simulink subsystem "INDI_Controller_PQR"  (R2023b)
settings: Solver=VariableStepAuto  StartTime=0.0  StopTime=10.0  RelTol=1e-3
undefined symbols (not defined in the file): controlDeflections, dataBase, deltaLEF
libraries: aerolibutil x1, simulink_extras x1
settings Model: Creator=cyber  LastModifiedBy=cyber

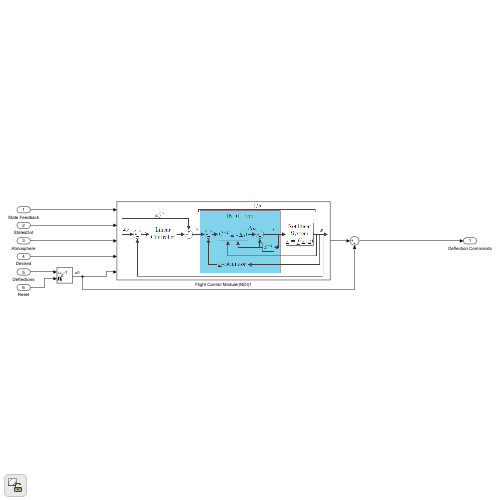
[thumbnail: Simulink's stored preview of the top-level diagram]
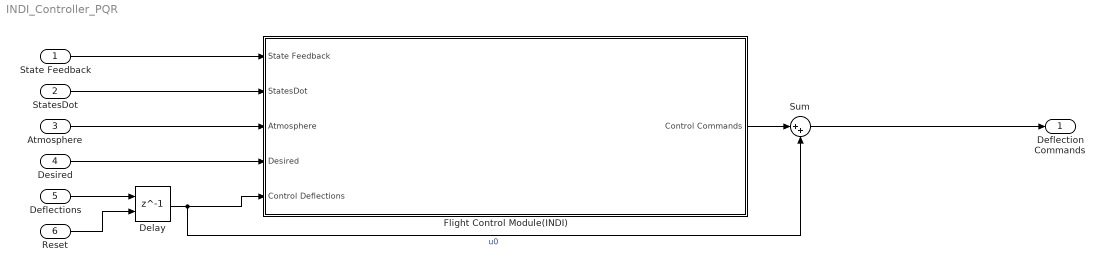
== system INDI_Controller_PQR ==
  State Feedback : Inport
  StatesDot : Inport  Port=2
  Atmosphere : Inport  Port=3
  Desired : Inport  Port=4
  Deflections : Inport  Port=5
  Reset : Inport  Port=6
  Delay : Delay  DelayLength=1  InitialCondition=[controlDeflections(1); controlDeflections(2); controlDeflections(3); controlDeflections(4); deltaLEF; 0]  ExternalReset=Either
      settings: InputPortMap=u0,r5
  Flight Control Module(INDI) : Subsystem
      mask Display: image('INDI.png'); % Use "Edit Image" on toolstrip to change.
  Sum : Sum  Inputs=|++
  Deflection Commands : Outport
  wires:
  Sum/1 -> Deflection Commands/1
  Flight Control Module(INDI)/1(Control Commands) -> Sum/1
  Reset/1 -> Delay/2
  Delay/1 -> Flight Control Module(INDI)/5(Control Deflections), Sum/2  "u0"
  Atmosphere/1 -> Flight Control Module(INDI)/3(Atmosphere)
  StatesDot/1 -> Flight Control Module(INDI)/2(StatesDot)
  State Feedback/1 -> Flight Control Module(INDI)/1(State Feedback)
  Deflections/1 -> Delay/1
  Desired/1 -> Flight Control Module(INDI)/4(Desired)

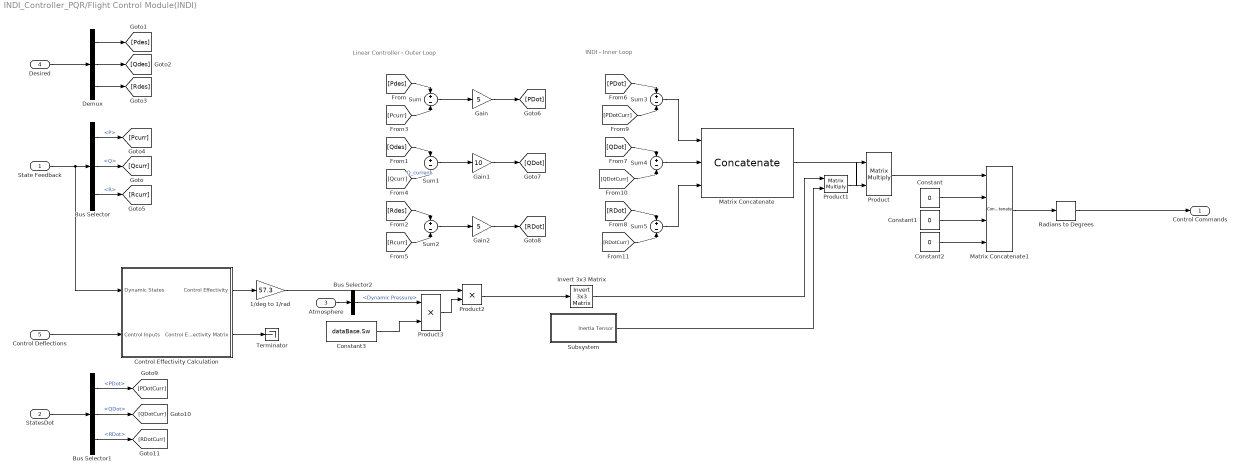
== system INDI_Controller_PQR/Flight Control Module(INDI) ==
  note: INDI - Inner Loop
  note: Linear Controller - Outer Loop
  State Feedback : Inport
  StatesDot : Inport  Port=2
  Atmosphere : Inport  Port=3
  Desired : Inport  Port=4
  Control Deflections : Inport  Port=5
  1/deg to 1/rad : Gain  Gain=57.3
  Bus Selector : BusSelector  OutputSignals=P,Q,R
  Bus Selector1 : BusSelector  OutputSignals=PDot,QDot,RDot
  Bus Selector2 : BusSelector  OutputSignals=Dynamic Pressure
  Constant : Constant  Value=0
  Constant1 : Constant  Value=0
  Constant2 : Constant  Value=0
  Constant3 : Constant  Value=dataBase.Sw
  Control Effectivity Calculation : Subsystem
      mask Display: image('F16.PNG'); % Use "Edit Image" on toolstrip to change.
  Demux : Demux  Outputs=3
  Gain : Gain  Gain=5
  Gain1 : Gain  Gain=10
  Gain2 : Gain  Gain=5
  Invert 3x3 Matrix : aerolibutil/Invert  3x3 Matrix
  Matrix Concatenate : Concatenate  NumInputs=3  Mode=Multidimensional array
  Matrix Concatenate1 : Concatenate  NumInputs=4  Mode=Multidimensional array
  Product : Product  Multiplication=Matrix(*)
  Product1 : Product  Multiplication=Matrix(*)
  Product2 : Product
  Product3 : Product
  Radians to Degrees : simulink_extras/Transformations/Radians to Degrees
  Subsystem : Subsystem
  Sum{,1..5} (6 alike) : Sum  Inputs=+|-
  Terminator : Terminator
  Control Commands : Outport
  wires:
  State Feedback/1 -> Control Effectivity Calculation/1(Dynamic States), Bus Selector/1
  Bus Selector/2 -> [Qcurr]  "<Q>"
  Desired/1 -> Demux/1
  Demux/1 -> [Pdes]
  Demux/2 -> [Qdes]
  Demux/3 -> [Rdes]
  Control Deflections/1 -> Control Effectivity Calculation/2(Control Inputs)
  Bus Selector/1 -> [Pcurr]  "<P>"
  Bus Selector/3 -> [Rcurr]  "<R>"
  [Pdes] -> Sum/1
  [Pcurr] -> Sum/2
  Sum/1 -> Gain/1
  [Qdes] -> Sum1/1
  [Qcurr] -> Sum1/2  "Q_current"
  Sum1/1 -> Gain1/1
  [Rdes] -> Sum2/1
  [Rcurr] -> Sum2/2
  Sum2/1 -> Gain2/1
  Gain/1 -> [PDot]
  Gain1/1 -> [QDot]
  Gain2/1 -> [RDot]
  StatesDot/1 -> Bus Selector1/1
  [PDot] -> Sum3/1
  [PDotCurr] -> Sum3/2
  [QDot] -> Sum4/1
  [QDotCurr] -> Sum4/2
  [RDot] -> Sum5/1
  [RDotCurr] -> Sum5/2
  Sum3/1 -> Matrix Concatenate/1
  Sum4/1 -> Matrix Concatenate/2
  Sum5/1 -> Matrix Concatenate/3
  Matrix Concatenate/1 -> Product/2
  Control Effectivity Calculation/1(Control Effectivity) -> 1/deg to 1/rad/1
  Product1/1 -> Product/1
  Constant/1 -> Matrix Concatenate1/2
  Constant1/1 -> Matrix Concatenate1/3
  Constant2/1 -> Matrix Concatenate1/4
  Matrix Concatenate1/1 -> Radians to Degrees/1
  Product/1 -> Matrix Concatenate1/1
  Radians to Degrees/1 -> Control Commands/1
  Bus Selector1/3 -> [RDotCurr]  "<RDot>"
  Bus Selector1/2 -> [QDotCurr]  "<QDot>"
  Bus Selector1/1 -> [PDotCurr]  "<PDot>"
  1/deg to 1/rad/1 -> Product2/1
  Product2/1 -> Invert 3x3 Matrix/1
  Atmosphere/1 -> Bus Selector2/1
  Product3/1 -> Product2/2
  Constant3/1 -> Product3/2
  Invert 3x3 Matrix/1 -> Product1/1
  Subsystem/1(Inertia Tensor) -> Product1/2
  Bus Selector2/1 -> Product3/1  "<Dynamic Pressure>"
  Control Effectivity Calculation/2(Control Effectivity Matrix) -> Terminator/1

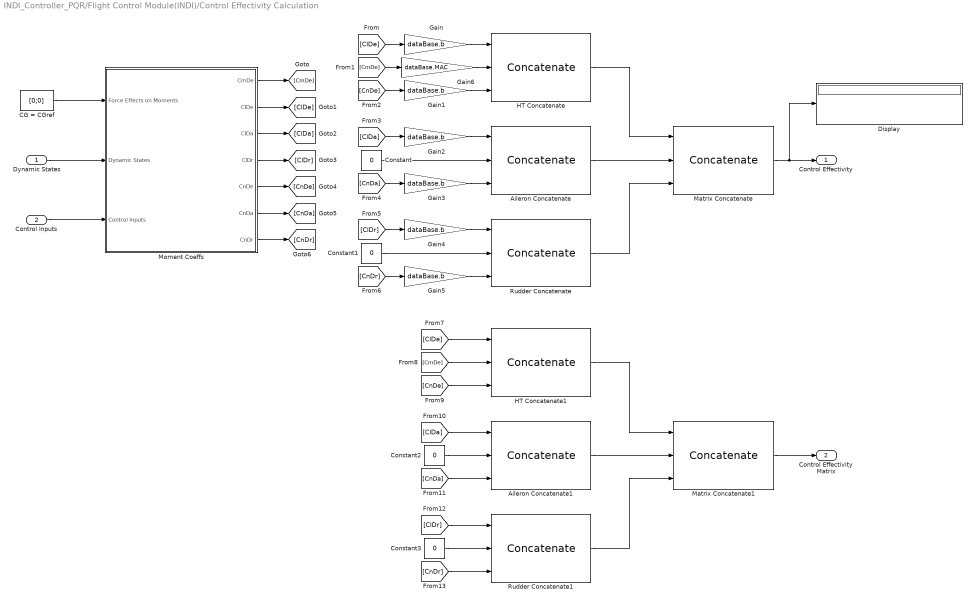
== system INDI_Controller_PQR/Flight Control Module(INDI)/Control Effectivity Calculation ==
  Dynamic States : Inport
  Control Inputs : Inport  Port=2
  Aileron Concatenate : Concatenate  NumInputs=3  Mode=Multidimensional array
  Aileron Concatenate1 : Concatenate  NumInputs=3  Mode=Multidimensional array
  CG = CGref : Constant  Value=[0;0]
  Constant{,1..3} (4 alike) : Constant  Value=0
  Display : Display
  Gain{,1..5} (6 alike) : Gain  Gain=dataBase.b
  Gain6 : Gain  Gain=dataBase.MAC
  HT Concatenate : Concatenate  NumInputs=3  Mode=Multidimensional array
  HT Concatenate1 : Concatenate  NumInputs=3  Mode=Multidimensional array
  Matrix Concatenate : Concatenate  NumInputs=3  Mode=Multidimensional array  ConcatenateDimension=2
  Matrix Concatenate1 : Concatenate  NumInputs=3  Mode=Multidimensional array  ConcatenateDimension=2
  Moment Coeffs : Subsystem
  Rudder Concatenate : Concatenate  NumInputs=3  Mode=Multidimensional array
  Rudder Concatenate1 : Concatenate  NumInputs=3  Mode=Multidimensional array
  Control Effectivity : Outport
  Control Effectivity Matrix : Outport  Port=2
  wires:
  Dynamic States/1 -> Moment Coeffs/2(Dynamic States)
  Control Inputs/1 -> Moment Coeffs/3(Control Inputs)
  CG = CGref/1 -> Moment Coeffs/1(Force Effects on Moments)
  Moment Coeffs/1(" CmDe") -> [CmDe]
  Moment Coeffs/2(" ClDe") -> [ClDe]
  Moment Coeffs/3(" ClDa") -> [ClDa]
  Moment Coeffs/4(" ClDr") -> [ClDr]
  Moment Coeffs/5(CnDe) -> [CnDe]
  Moment Coeffs/6(CnDa) -> [CnDa]
  Moment Coeffs/7(CnDr) -> [CnDr]
  HT Concatenate/1 -> Matrix Concatenate/1
  Aileron Concatenate/1 -> Matrix Concatenate/2
  Rudder Concatenate/1 -> Matrix Concatenate/3
  [ClDe] -> Gain/1
  [CmDe] -> Gain6/1
  [CnDe] -> Gain1/1
  [ClDa] -> Gain2/1
  Constant/1 -> Aileron Concatenate/2
  [CnDa] -> Gain3/1
  [ClDr] -> Gain4/1
  [CnDr] -> Gain5/1
  Constant1/1 -> Rudder Concatenate/2
  Matrix Concatenate/1 -> Display/1, Control Effectivity/1
  Gain/1 -> HT Concatenate/1
  Gain1/1 -> HT Concatenate/3
  Gain2/1 -> Aileron Concatenate/1
  Gain3/1 -> Aileron Concatenate/3
  Gain4/1 -> Rudder Concatenate/1
  Gain5/1 -> Rudder Concatenate/3
  Gain6/1 -> HT Concatenate/2
  [CmDe] -> HT Concatenate1/2
  [ClDe] -> HT Concatenate1/1
  [CnDa] -> Aileron Concatenate1/3
  [CnDe] -> HT Concatenate1/3
  [ClDa] -> Aileron Concatenate1/1
  Rudder Concatenate1/1 -> Matrix Concatenate1/3
  Matrix Concatenate1/1 -> Control Effectivity Matrix/1
  [ClDr] -> Rudder Concatenate1/1
  HT Concatenate1/1 -> Matrix Concatenate1/1
  [CnDr] -> Rudder Concatenate1/3
  Aileron Concatenate1/1 -> Matrix Concatenate1/2
  Constant2/1 -> Aileron Concatenate1/2
  Constant3/1 -> Rudder Concatenate1/2

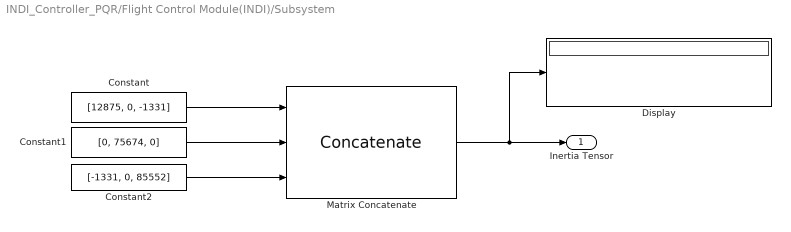
== system INDI_Controller_PQR/Flight Control Module(INDI)/Subsystem ==
  Constant : Constant  Value=[12875, 0, -1331]
  Constant1 : Constant  Value=[0, 75674, 0]
  Constant2 : Constant  Value=[-1331, 0, 85552]
  Display : Display
  Matrix Concatenate : Concatenate  NumInputs=3  Mode=Multidimensional array  ConcatenateDimension=2
  Inertia Tensor : Outport
  wires:
  Constant/1 -> Matrix Concatenate/1
  Constant2/1 -> Matrix Concatenate/3
  Constant1/1 -> Matrix Concatenate/2
  Matrix Concatenate/1 -> Display/1, Inertia Tensor/1

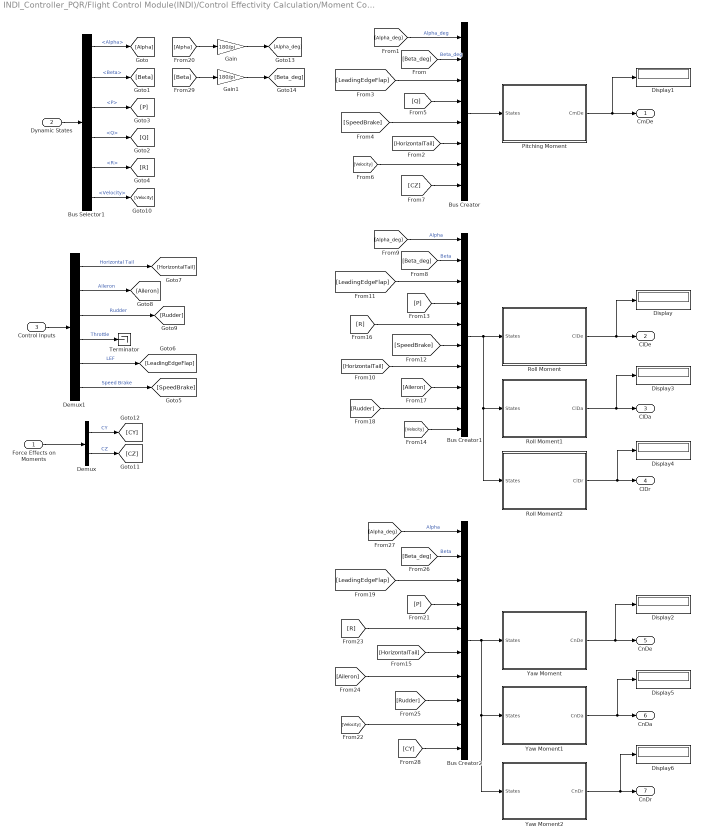
== system INDI_Controller_PQR/Flight Control Module(INDI)/Control Effectivity Calculation/Moment Coeffs ==
  Force Effects on Moments : Inport
  Dynamic States : Inport  Port=2
  Control Inputs : Inport  Port=3
  Bus Creator : BusCreator  Inputs=8
  Bus Creator1 : BusCreator  Inputs=10
  Bus Creator2 : BusCreator  Inputs=10
  Bus Selector1 : BusSelector  OutputSignals=Alpha,Beta,P,Q,R,Velocity
  Demux : Demux  Outputs=2
  Demux1 : Demux  Outputs=6
  Display{,1..6} (7 alike) : Display
  Gain : Gain  Gain=180/pi
  Gain1 : Gain  Gain=180/pi
  Pitching Moment : Subsystem
  Roll Moment : Subsystem
  Roll Moment1 : Subsystem
  Roll Moment2 : Subsystem
  Terminator : Terminator
  Yaw Moment : Subsystem
  Yaw Moment1 : Subsystem
  Yaw Moment2 : Subsystem
  " CmDe" : Outport
  " ClDe" : Outport  Port=2
  " ClDa" : Outport  Port=3
  " ClDr" : Outport  Port=4
  CnDe : Outport  Port=5
  CnDa : Outport  Port=6
  CnDr : Outport  Port=7
  wires:
  Pitching Moment/1(CmDe) -> Display1/1, " CmDe"/1
  Bus Creator/1 -> Pitching Moment/1(States)
  [SpeedBrake] -> Bus Creator/5
  [LeadingEdgeFlap] -> Bus Creator/3
  [Q] -> Bus Creator/4
  [HorizontalTail] -> Bus Creator/6
  [Velocity] -> Bus Creator/7
  [CZ] -> Bus Creator/8
  Force Effects on Moments/1 -> Demux/1
  Demux/1 -> [CY]  "CY"
  Demux/2 -> [CZ]  "CZ"
  [P] -> Bus Creator1/4
  [LeadingEdgeFlap] -> Bus Creator1/3
  Roll Moment/1(ClDe) -> Display/1, " ClDe"/1
  [Velocity] -> Bus Creator1/10
  [R] -> Bus Creator1/5
  [SpeedBrake] -> Bus Creator1/6
  [HorizontalTail] -> Bus Creator1/7
  [Aileron] -> Bus Creator1/8
  [Rudder] -> Bus Creator1/9
  [Rudder] -> Bus Creator2/8
  [Aileron] -> Bus Creator2/7
  [HorizontalTail] -> Bus Creator2/6
  [R] -> Bus Creator2/5
  [Velocity] -> Bus Creator2/9
  [LeadingEdgeFlap] -> Bus Creator2/3
  [P] -> Bus Creator2/4
  Bus Creator2/1 -> Yaw Moment2/1(States), Yaw Moment1/1(States), Yaw Moment/1(States)
  Bus Selector1/4 -> [Q]  "<Q>"
  Demux1/1 -> [HorizontalTail]  "Horizontal Tail"
  Control Inputs/1 -> Demux1/1
  Demux1/6 -> [SpeedBrake]  "Speed Brake"
  Demux1/2 -> [Aileron]  "Aileron"
  Bus Selector1/6 -> [Velocity]  "<Velocity>"
  Bus Selector1/3 -> [P]  "<P>"
  Bus Selector1/2 -> [Beta]  "<Beta>"
  Demux1/3 -> [Rudder]  "Rudder"
  Bus Selector1/5 -> [R]  "<R>"
  Demux1/5 -> [LeadingEdgeFlap]  "LEF"
  Dynamic States/1 -> Bus Selector1/1
  Bus Selector1/1 -> [Alpha]  "<Alpha>"
  Bus Creator1/1 -> Roll Moment2/1(States), Roll Moment1/1(States), Roll Moment/1(States)
  Gain1/1 -> [Beta_deg]
  [Beta] -> Gain1/1
  [Alpha] -> Gain/1
  Gain/1 -> [Alpha_deg]
  [Alpha_deg] -> Bus Creator/1  "Alpha_deg"
  [Beta_deg] -> Bus Creator/2  "Beta_deg"
  [Alpha_deg] -> Bus Creator1/1  "Alpha"
  [Beta_deg] -> Bus Creator1/2  "Beta"
  [Alpha_deg] -> Bus Creator2/1  "Alpha"
  [Beta_deg] -> Bus Creator2/2  "Beta"
  [CY] -> Bus Creator2/10
  Roll Moment1/1(ClDa) -> Display3/1, " ClDa"/1
  Roll Moment2/1(ClDr) -> Display4/1, " ClDr"/1
  Yaw Moment/1(CnDe) -> CnDe/1, Display2/1
  Yaw Moment1/1(CnDa) -> Display5/1, CnDa/1
  Yaw Moment2/1(CnDr) -> Display6/1, CnDr/1
  Demux1/4 -> Terminator/1  "Throttle"

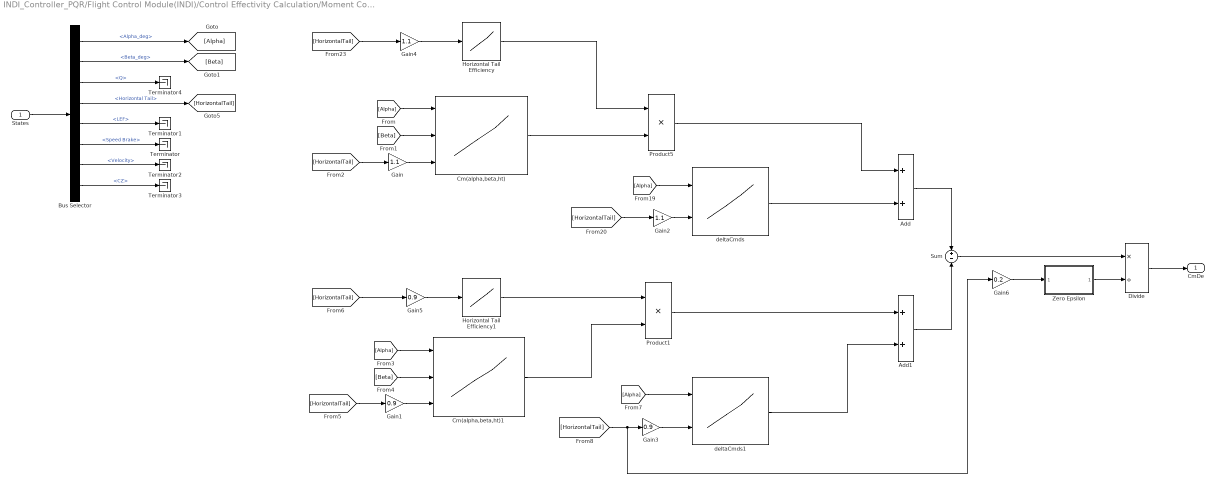
== system INDI_Controller_PQR/Flight Control Module(INDI)/Control Effectivity Calculation/Moment Coeffs/Pitching Moment ==
  States : Inport
  Add : Sum
  Add1 : Sum
  Bus Selector : BusSelector  OutputSignals=Alpha_deg,Beta_deg,Q,Horizontal Tail,LEF,Speed Brake,Velocity,CZ
  Cm(alpha,beta,ht) : Lookup_n-D  NumberOfTableDimensions=3  BreakpointsForDimension1=dataBase.f16_AerodynamicData.BP.Cm.Cm.alpha  BreakpointsForDimension2=dataBase.f16_AerodynamicData.BP.Cm.Cm.beta  BreakpointsForDimension3=dataBase.f16_AerodynamicData.BP.Cm.Cm.dHT  Table=dataBase.f16_AerodynamicData.data.Cm.Cm  ExtrapMethod=Clip  InternalRulePriority=Speed  RndMeth=Simplest
      settings: InputPortMap=u0,u1,u2
  Cm(alpha,beta,ht)1 : Lookup_n-D  NumberOfTableDimensions=3  BreakpointsForDimension1=dataBase.f16_AerodynamicData.BP.Cm.Cm.alpha  BreakpointsForDimension2=dataBase.f16_AerodynamicData.BP.Cm.Cm.beta  BreakpointsForDimension3=dataBase.f16_AerodynamicData.BP.Cm.Cm.dHT  Table=dataBase.f16_AerodynamicData.data.Cm.Cm  ExtrapMethod=Clip  InternalRulePriority=Speed  RndMeth=Simplest
      settings: InputPortMap=u0,u1,u2
  Divide : Product  Inputs=*/
  Gain : Gain  Gain=1.1
  Gain1 : Gain  Gain=0.9
  Gain2 : Gain  Gain=1.1
  Gain3 : Gain  Gain=0.9
  Gain4 : Gain  Gain=1.1
  Gain5 : Gain  Gain=0.9
  Gain6 : Gain  Gain=0.2
  Horizontal Tail Efficiency : Lookup_n-D  NumberOfTableDimensions=1  BreakpointsForDimension1=dataBase.f16_AerodynamicData.BP.Cm.n_dHT.dHT  Table=dataBase.f16_AerodynamicData.data.Cm.n_dHT  ExtrapMethod=Clip  InternalRulePriority=Speed  RndMeth=Simplest
  Horizontal Tail Efficiency1 : Lookup_n-D  NumberOfTableDimensions=1  BreakpointsForDimension1=dataBase.f16_AerodynamicData.BP.Cm.n_dHT.dHT  Table=dataBase.f16_AerodynamicData.data.Cm.n_dHT  ExtrapMethod=Clip  InternalRulePriority=Speed  RndMeth=Simplest
  Product1 : Product
  Product5 : Product
  Sum : Sum  Inputs=+|-
  Terminator{,1..4} (5 alike) : Terminator
  Zero Epsilon : Subsystem  ReferencedSubsystem=Zero_Epsilon
  deltaCmds : Lookup_n-D  BreakpointsForDimension1=dataBase.f16_AerodynamicData.BP.Cm.deltaCmds.alpha  BreakpointsForDimension2=dataBase.f16_AerodynamicData.BP.Cm.deltaCmds.dHT  Table=dataBase.f16_AerodynamicData.data.Cm.deltaCmds  ExtrapMethod=Clip  InternalRulePriority=Speed  RndMeth=Simplest
      settings: InputPortMap=u0,u1
  deltaCmds1 : Lookup_n-D  BreakpointsForDimension1=dataBase.f16_AerodynamicData.BP.Cm.deltaCmds.alpha  BreakpointsForDimension2=dataBase.f16_AerodynamicData.BP.Cm.deltaCmds.dHT  Table=dataBase.f16_AerodynamicData.data.Cm.deltaCmds  ExtrapMethod=Clip  InternalRulePriority=Speed  RndMeth=Simplest
      settings: InputPortMap=u0,u1
  CmDe : Outport
  wires:
  Zero Epsilon/1 -> Divide/2
  Gain6/1 -> Zero Epsilon/1
  [Alpha] -> Cm(alpha,beta,ht)/1
  States/1 -> Bus Selector/1
  [Beta] -> Cm(alpha,beta,ht)/2
  [Alpha] -> deltaCmds/1
  Product5/1 -> Add/1
  Cm(alpha,beta,ht)/1 -> Product5/2
  Horizontal Tail Efficiency/1 -> Product5/1
  Bus Selector/1 -> [Alpha]  "<Alpha_deg>"
  Bus Selector/2 -> [Beta]  "<Beta_deg>"
  Bus Selector/3 -> Terminator4/1  "<Q>"
  Bus Selector/4 -> [HorizontalTail]  "<Horizontal Tail>"
  Bus Selector/5 -> Terminator1/1  "<LEF>"
  Bus Selector/6 -> Terminator/1  "<Speed Brake>"
  Bus Selector/7 -> Terminator2/1  "<Velocity>"
  Bus Selector/8 -> Terminator3/1  "<CZ>"
  [HorizontalTail] -> Gain/1
  Gain/1 -> Cm(alpha,beta,ht)/3
  [HorizontalTail] -> Gain2/1
  Gain2/1 -> deltaCmds/2
  Add/1 -> Sum/1
  [HorizontalTail] -> Gain1/1
  Gain1/1 -> Cm(alpha,beta,ht)1/3
  [Beta] -> Cm(alpha,beta,ht)1/2
  Horizontal Tail Efficiency1/1 -> Product1/1
  [Alpha] -> Cm(alpha,beta,ht)1/1
  Cm(alpha,beta,ht)1/1 -> Product1/2
  [HorizontalTail] -> Gain3/1, Gain6/1
  Gain3/1 -> deltaCmds1/2
  [Alpha] -> deltaCmds1/1
  Product1/1 -> Add1/1
  deltaCmds1/1 -> Add1/2
  Add1/1 -> Sum/2
  deltaCmds/1 -> Add/2
  Sum/1 -> Divide/1
  Divide/1 -> CmDe/1
  [HorizontalTail] -> Gain4/1
  Gain4/1 -> Horizontal Tail Efficiency/1
  [HorizontalTail] -> Gain5/1
  Gain5/1 -> Horizontal Tail Efficiency1/1

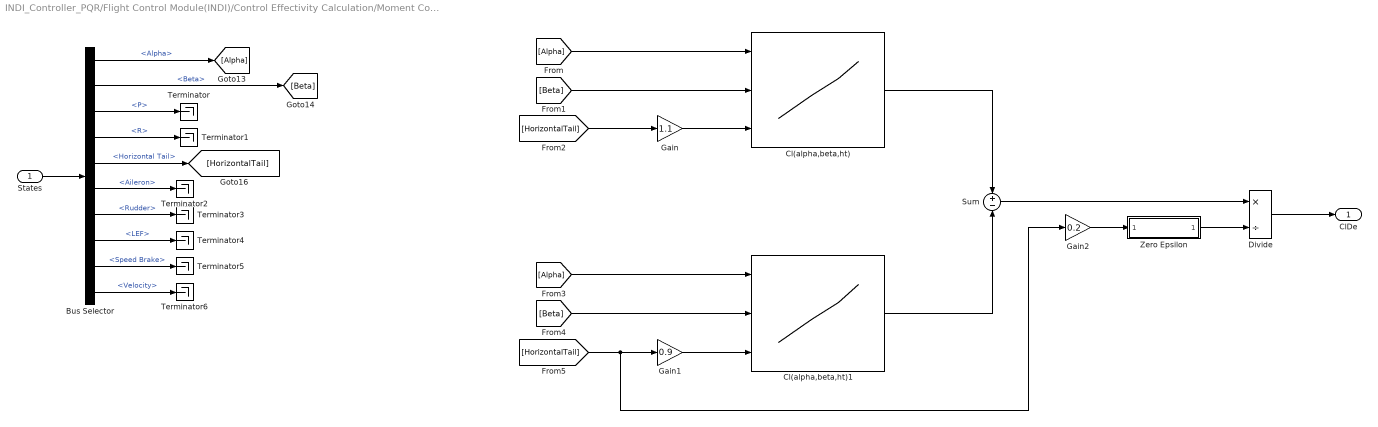
== system INDI_Controller_PQR/Flight Control Module(INDI)/Control Effectivity Calculation/Moment Coeffs/Roll Moment ==
  States : Inport
  Bus Selector : BusSelector  OutputSignals=Alpha,Beta,P,R,Horizontal Tail,Aileron,Rudder,LEF,Speed Brake,Velocity
  Cl(alpha,beta,ht) : Lookup_n-D  NumberOfTableDimensions=3  BreakpointsForDimension1=dataBase.f16_AerodynamicData.BP.Cl.Cl.alpha  BreakpointsForDimension2=dataBase.f16_AerodynamicData.BP.Cl.Cl.beta  BreakpointsForDimension3=dataBase.f16_AerodynamicData.BP.Cl.Cl.dHT  Table=dataBase.f16_AerodynamicData.data.Cl.Cl  ExtrapMethod=Clip  InternalRulePriority=Speed  RndMeth=Simplest
      settings: InputPortMap=u0,u1,u2
  Cl(alpha,beta,ht)1 : Lookup_n-D  NumberOfTableDimensions=3  BreakpointsForDimension1=dataBase.f16_AerodynamicData.BP.Cl.Cl.alpha  BreakpointsForDimension2=dataBase.f16_AerodynamicData.BP.Cl.Cl.beta  BreakpointsForDimension3=dataBase.f16_AerodynamicData.BP.Cl.Cl.dHT  Table=dataBase.f16_AerodynamicData.data.Cl.Cl  ExtrapMethod=Clip  InternalRulePriority=Speed  RndMeth=Simplest
      settings: InputPortMap=u0,u1,u2
  Divide : Product  Inputs=*/
  Gain : Gain  Gain=1.1
  Gain1 : Gain  Gain=0.9
  Gain2 : Gain  Gain=0.2
  Sum : Sum  Inputs=+|-
  Terminator{,1..6} (7 alike) : Terminator
  Zero Epsilon : Subsystem  ReferencedSubsystem=Zero_Epsilon
  ClDe : Outport
  wires:
  Zero Epsilon/1 -> Divide/2
  Gain2/1 -> Zero Epsilon/1
  Cl(alpha,beta,ht)/1 -> Sum/1
  [Alpha] -> Cl(alpha,beta,ht)/1
  [Beta] -> Cl(alpha,beta,ht)/2
  Bus Selector/5 -> [HorizontalTail]  "<Horizontal Tail>"
  States/1 -> Bus Selector/1
  Bus Selector/2 -> [Beta]  "<Beta>"
  Bus Selector/1 -> [Alpha]  "<Alpha>"
  [Alpha] -> Cl(alpha,beta,ht)1/1
  [Beta] -> Cl(alpha,beta,ht)1/2
  Cl(alpha,beta,ht)1/1 -> Sum/2
  [HorizontalTail] -> Gain/1
  Gain/1 -> Cl(alpha,beta,ht)/3
  [HorizontalTail] -> Gain2/1, Gain1/1
  Gain1/1 -> Cl(alpha,beta,ht)1/3
  Sum/1 -> Divide/1
  Divide/1 -> ClDe/1
  Bus Selector/3 -> Terminator/1  "<P>"
  Bus Selector/4 -> Terminator1/1  "<R>"
  Bus Selector/6 -> Terminator2/1  "<Aileron>"
  Bus Selector/7 -> Terminator3/1  "<Rudder>"
  Bus Selector/8 -> Terminator4/1  "<LEF>"
  Bus Selector/9 -> Terminator5/1  "<Speed Brake>"
  Bus Selector/10 -> Terminator6/1  "<Velocity>"

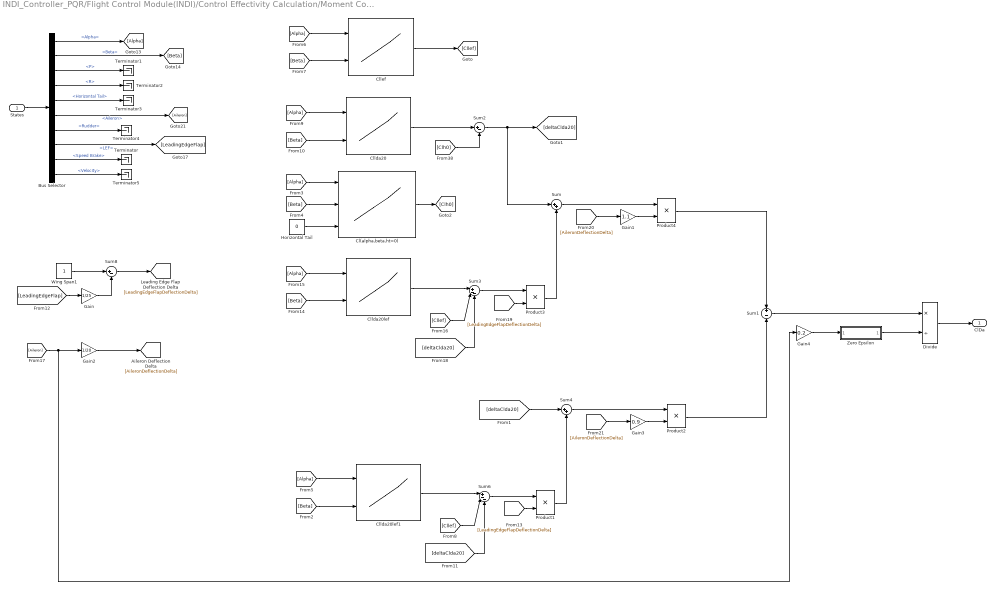
== system INDI_Controller_PQR/Flight Control Module(INDI)/Control Effectivity Calculation/Moment Coeffs/Roll Moment1 ==
  States : Inport
  Bus Selector : BusSelector  OutputSignals=Alpha,Beta,P,R,Horizontal Tail,Aileron,Rudder,LEF,Speed Brake,Velocity
  Cl(alpha,beta,ht=0) : Lookup_n-D  NumberOfTableDimensions=3  BreakpointsForDimension1=dataBase.f16_AerodynamicData.BP.Cl.Cl.alpha  BreakpointsForDimension2=dataBase.f16_AerodynamicData.BP.Cl.Cl.beta  BreakpointsForDimension3=dataBase.f16_AerodynamicData.BP.Cl.Cl.dHT  Table=dataBase.f16_AerodynamicData.data.Cl.Cl  ExtrapMethod=Clip  InternalRulePriority=Speed  RndMeth=Simplest
      settings: InputPortMap=u0,u1,u2
  Cllda20 : Lookup_n-D  BreakpointsForDimension1=dataBase.f16_AerodynamicData.BP.Cl.Clda20.alpha  BreakpointsForDimension2=dataBase.f16_AerodynamicData.BP.Cl.Clda20.beta  Table=dataBase.f16_AerodynamicData.data.Cl.Clda20  ExtrapMethod=Clip  InternalRulePriority=Speed  RndMeth=Simplest
      settings: InputPortMap=u0,u1
  Cllda20lef : Lookup_n-D  BreakpointsForDimension1=dataBase.f16_AerodynamicData.BP.Cl.Clda20lef.alpha  BreakpointsForDimension2=dataBase.f16_AerodynamicData.BP.Cl.Clda20lef.beta  Table=dataBase.f16_AerodynamicData.data.Cl.Clda20lef  ExtrapMethod=Clip  InternalRulePriority=Speed  RndMeth=Simplest
      settings: InputPortMap=u0,u1
  Cllda20lef1 : Lookup_n-D  BreakpointsForDimension1=dataBase.f16_AerodynamicData.BP.Cl.Clda20lef.alpha  BreakpointsForDimension2=dataBase.f16_AerodynamicData.BP.Cl.Clda20lef.beta  Table=dataBase.f16_AerodynamicData.data.Cl.Clda20lef  ExtrapMethod=Clip  InternalRulePriority=Speed  RndMeth=Simplest
      settings: InputPortMap=u0,u1
  Cllef : Lookup_n-D  BreakpointsForDimension1=dataBase.f16_AerodynamicData.BP.Cl.Cllef.alpha  BreakpointsForDimension2=dataBase.f16_AerodynamicData.BP.Cl.Cllef.beta  Table=dataBase.f16_AerodynamicData.data.Cl.Cllef  ExtrapMethod=Clip  InternalRulePriority=Speed  RndMeth=Simplest
      settings: InputPortMap=u0,u1
  Divide : Product  Inputs=*/
  Gain : Gain  Gain=1/25
  Gain1 : Gain  Gain=1.1
  Gain2 : Gain  Gain=1/20
  Gain3 : Gain  Gain=0.9
  Gain4 : Gain  Gain=0.2
  Horizontal Tail : Constant  Value=0
  Product{1..4} (4 alike) : Product
  Sum : Sum  Inputs=|++
  Sum1 : Sum  Inputs=+|-
  Sum2 : Sum  Inputs=|+-
  Sum3 : Sum  Inputs=|+--
  Sum4 : Sum  Inputs=|++
  Sum6 : Sum  Inputs=|+--
  Sum8 : Sum  Inputs=|+-
  Terminator{,1..5} (6 alike) : Terminator
  Wing Span1 : Constant
  Zero Epsilon : Subsystem  ReferencedSubsystem=Zero_Epsilon
  ClDa : Outport
  wires:
  Zero Epsilon/1 -> Divide/2
  Gain4/1 -> Zero Epsilon/1
  [Beta] -> Cllef/2
  [Alpha] -> Cllef/1
  Gain/1 -> Sum8/2
  [LeadingEdgeFlap] -> Gain/1
  [Aileron] -> Gain4/1, Gain2/1
  Gain2/1 -> [AileronDeflectionDelta]
  [Beta] -> Cl(alpha,beta,ht=0)/2
  Horizontal Tail/1 -> Cl(alpha,beta,ht=0)/3
  [Alpha] -> Cl(alpha,beta,ht=0)/1
  Cllef/1 -> [Cllef]
  Cl(alpha,beta,ht=0)/1 -> [Clh0]
  [Beta] -> Cllda20/2
  [Alpha] -> Cllda20/1
  Cllda20/1 -> Sum2/1
  Sum2/1 -> Sum/1, [deltaClda20]
  [Alpha] -> Cllda20lef/1
  [Beta] -> Cllda20lef/2
  Cllda20lef/1 -> Sum3/1
  [Cllef] -> Sum3/2
  [deltaClda20] -> Sum3/3
  [LeadingEdgeFlapDeflectionDelta] -> Product3/2
  Sum3/1 -> Product3/1
  Product3/1 -> Sum/2
  Sum/1 -> Product4/1
  Product4/1 -> Sum1/1
  [Clh0] -> Sum2/2
  Bus Selector/7 -> Terminator4/1  "<Rudder>"
  Bus Selector/3 -> Terminator1/1  "<P>"
  Bus Selector/5 -> Terminator3/1  "<Horizontal Tail>"
  States/1 -> Bus Selector/1
  Bus Selector/2 -> [Beta]  "<Beta>"
  Bus Selector/1 -> [Alpha]  "<Alpha>"
  Bus Selector/6 -> [Aileron]  "<Aileron>"
  Bus Selector/8 -> [LeadingEdgeFlap]  "<LEF>"
  Bus Selector/4 -> Terminator2/1  "<R>"
  Bus Selector/9 -> Terminator/1  "<Speed Brake>"
  Wing Span1/1 -> Sum8/1
  Sum8/1 -> [LeadingEdgeFlapDeflectionDelta]
  [AileronDeflectionDelta] -> Gain1/1
  Gain1/1 -> Product4/2
  [Beta] -> Cllda20lef1/2
  [deltaClda20] -> Sum6/3
  [LeadingEdgeFlapDeflectionDelta] -> Product1/2
  Product1/1 -> Sum4/2
  [Cllef] -> Sum6/2
  Cllda20lef1/1 -> Sum6/1
  Sum4/1 -> Product2/1
  [Alpha] -> Cllda20lef1/1
  Sum6/1 -> Product1/1
  [AileronDeflectionDelta] -> Gain3/1
  Gain3/1 -> Product2/2
  [deltaClda20] -> Sum4/1
  Product2/1 -> Sum1/2
  Sum1/1 -> Divide/1
  Divide/1 -> ClDa/1
  Bus Selector/10 -> Terminator5/1  "<Velocity>"

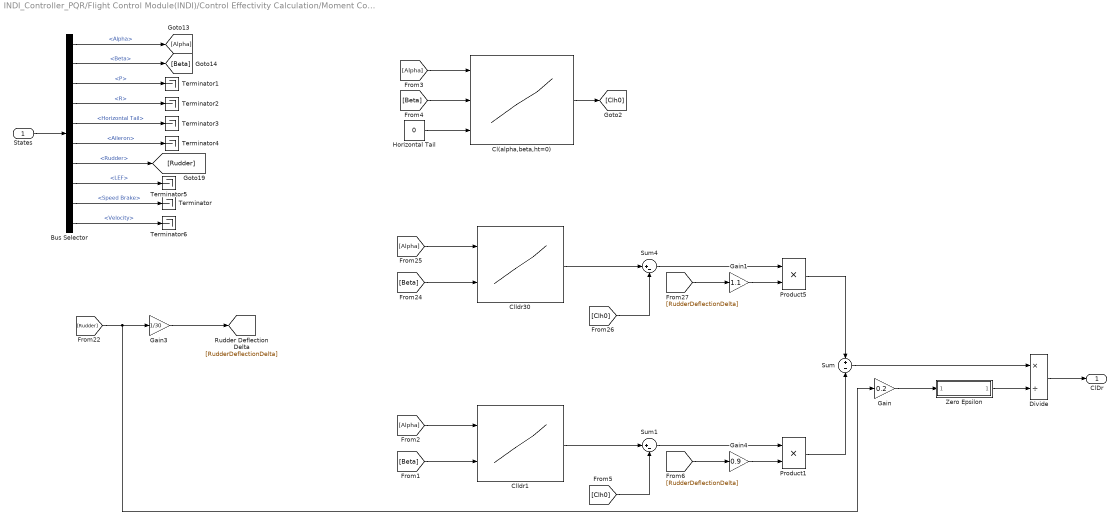
== system INDI_Controller_PQR/Flight Control Module(INDI)/Control Effectivity Calculation/Moment Coeffs/Roll Moment2 ==
  States : Inport
  Bus Selector : BusSelector  OutputSignals=Alpha,Beta,P,R,Horizontal Tail,Aileron,Rudder,LEF,Speed Brake,Velocity
  Cl(alpha,beta,ht=0) : Lookup_n-D  NumberOfTableDimensions=3  BreakpointsForDimension1=dataBase.f16_AerodynamicData.BP.Cl.Cl.alpha  BreakpointsForDimension2=dataBase.f16_AerodynamicData.BP.Cl.Cl.beta  BreakpointsForDimension3=dataBase.f16_AerodynamicData.BP.Cl.Cl.dHT  Table=dataBase.f16_AerodynamicData.data.Cl.Cl  ExtrapMethod=Clip  InternalRulePriority=Speed  RndMeth=Simplest
      settings: InputPortMap=u0,u1,u2
  Clldr1 : Lookup_n-D  BreakpointsForDimension1=dataBase.f16_AerodynamicData.BP.Cl.Cldr30.alpha  BreakpointsForDimension2=dataBase.f16_AerodynamicData.BP.Cl.Cldr30.beta  Table=dataBase.f16_AerodynamicData.data.Cl.Cldr30  ExtrapMethod=Clip  InternalRulePriority=Speed  RndMeth=Simplest
      settings: InputPortMap=u0,u1
  Clldr30 : Lookup_n-D  BreakpointsForDimension1=dataBase.f16_AerodynamicData.BP.Cl.Cldr30.alpha  BreakpointsForDimension2=dataBase.f16_AerodynamicData.BP.Cl.Cldr30.beta  Table=dataBase.f16_AerodynamicData.data.Cl.Cldr30  ExtrapMethod=Clip  InternalRulePriority=Speed  RndMeth=Simplest
      settings: InputPortMap=u0,u1
  Divide : Product  Inputs=*/
  Gain : Gain  Gain=0.2
  Gain1 : Gain  Gain=1.1
  Gain3 : Gain  Gain=1/30
  Gain4 : Gain  Gain=0.9
  Horizontal Tail : Constant  Value=0
  Product1 : Product
  Product5 : Product
  Sum : Sum  Inputs=+|-
  Sum1 : Sum  Inputs=|+-
  Sum4 : Sum  Inputs=|+-
  Terminator{,1..6} (7 alike) : Terminator
  Zero Epsilon : Subsystem  ReferencedSubsystem=Zero_Epsilon
  ClDr : Outport
  wires:
  Zero Epsilon/1 -> Divide/2
  Gain/1 -> Zero Epsilon/1
  Gain3/1 -> [RudderDeflectionDelta]
  [Rudder] -> Gain/1, Gain3/1
  [Beta] -> Cl(alpha,beta,ht=0)/2
  Horizontal Tail/1 -> Cl(alpha,beta,ht=0)/3
  [Alpha] -> Cl(alpha,beta,ht=0)/1
  Cl(alpha,beta,ht=0)/1 -> [Clh0]
  [Alpha] -> Clldr30/1
  [Beta] -> Clldr30/2
  Clldr30/1 -> Sum4/1
  [Clh0] -> Sum4/2
  Sum4/1 -> Product5/1
  Bus Selector/7 -> [Rudder]  "<Rudder>"
  Bus Selector/3 -> Terminator1/1  "<P>"
  Bus Selector/5 -> Terminator3/1  "<Horizontal Tail>"
  States/1 -> Bus Selector/1
  Bus Selector/2 -> [Beta]  "<Beta>"
  Bus Selector/10 -> Terminator6/1  "<Velocity>"
  Bus Selector/1 -> [Alpha]  "<Alpha>"
  Bus Selector/6 -> Terminator4/1  "<Aileron>"
  Bus Selector/8 -> Terminator5/1  "<LEF>"
  Bus Selector/4 -> Terminator2/1  "<R>"
  Bus Selector/9 -> Terminator/1  "<Speed Brake>"
  [RudderDeflectionDelta] -> Gain1/1
  Gain1/1 -> Product5/2
  Product5/1 -> Sum/1
  Gain4/1 -> Product1/2
  Sum1/1 -> Product1/1
  [Beta] -> Clldr1/2
  Clldr1/1 -> Sum1/1
  [Clh0] -> Sum1/2
  [RudderDeflectionDelta] -> Gain4/1
  [Alpha] -> Clldr1/1
  Product1/1 -> Sum/2
  Sum/1 -> Divide/1
  Divide/1 -> ClDr/1

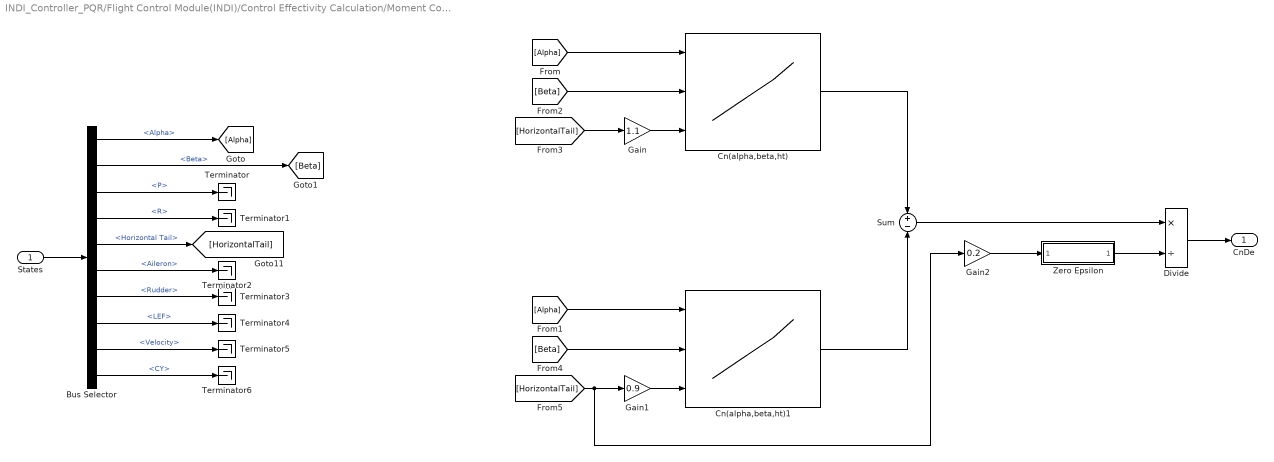
== system INDI_Controller_PQR/Flight Control Module(INDI)/Control Effectivity Calculation/Moment Coeffs/Yaw Moment ==
  States : Inport
  Bus Selector : BusSelector  OutputSignals=Alpha,Beta,P,R,Horizontal Tail,Aileron,Rudder,LEF,Velocity,CY
  Cn(alpha,beta,ht) : Lookup_n-D  NumberOfTableDimensions=3  BreakpointsForDimension1=dataBase.f16_AerodynamicData.BP.Cn.Cn.alpha  BreakpointsForDimension2=dataBase.f16_AerodynamicData.BP.Cn.Cn.beta  BreakpointsForDimension3=dataBase.f16_AerodynamicData.BP.Cn.Cn.dHT  Table=dataBase.f16_AerodynamicData.data.Cn.Cn  ExtrapMethod=Clip  InternalRulePriority=Speed  RndMeth=Simplest
      settings: InputPortMap=u0,u1,u2
  Cn(alpha,beta,ht)1 : Lookup_n-D  NumberOfTableDimensions=3  BreakpointsForDimension1=dataBase.f16_AerodynamicData.BP.Cn.Cn.alpha  BreakpointsForDimension2=dataBase.f16_AerodynamicData.BP.Cn.Cn.beta  BreakpointsForDimension3=dataBase.f16_AerodynamicData.BP.Cn.Cn.dHT  Table=dataBase.f16_AerodynamicData.data.Cn.Cn  ExtrapMethod=Clip  InternalRulePriority=Speed  RndMeth=Simplest
      settings: InputPortMap=u0,u1,u2
  Divide : Product  Inputs=*/
  Gain : Gain  Gain=1.1
  Gain1 : Gain  Gain=0.9
  Gain2 : Gain  Gain=0.2
  Sum : Sum  Inputs=+|-
  Terminator{,1..6} (7 alike) : Terminator
  Zero Epsilon : Subsystem  ReferencedSubsystem=Zero_Epsilon
  CnDe : Outport
  wires:
  Zero Epsilon/1 -> Divide/2
  Gain2/1 -> Zero Epsilon/1
  States/1 -> Bus Selector/1
  [Alpha] -> Cn(alpha,beta,ht)/1
  [Beta] -> Cn(alpha,beta,ht)/2
  Cn(alpha,beta,ht)/1 -> Sum/1
  Bus Selector/1 -> [Alpha]  "<Alpha>"
  Bus Selector/2 -> [Beta]  "<Beta>"
  Bus Selector/4 -> Terminator1/1  "<R>"
  Bus Selector/3 -> Terminator/1  "<P>"
  Bus Selector/5 -> [HorizontalTail]  "<Horizontal Tail>"
  Bus Selector/6 -> Terminator2/1  "<Aileron>"
  [HorizontalTail] -> Gain/1
  Gain/1 -> Cn(alpha,beta,ht)/3
  [HorizontalTail] -> Gain2/1, Gain1/1
  Gain1/1 -> Cn(alpha,beta,ht)1/3
  [Alpha] -> Cn(alpha,beta,ht)1/1
  [Beta] -> Cn(alpha,beta,ht)1/2
  Cn(alpha,beta,ht)1/1 -> Sum/2
  Sum/1 -> Divide/1
  Divide/1 -> CnDe/1
  Bus Selector/7 -> Terminator3/1  "<Rudder>"
  Bus Selector/8 -> Terminator4/1  "<LEF>"
  Bus Selector/9 -> Terminator5/1  "<Velocity>"
  Bus Selector/10 -> Terminator6/1  "<CY>"

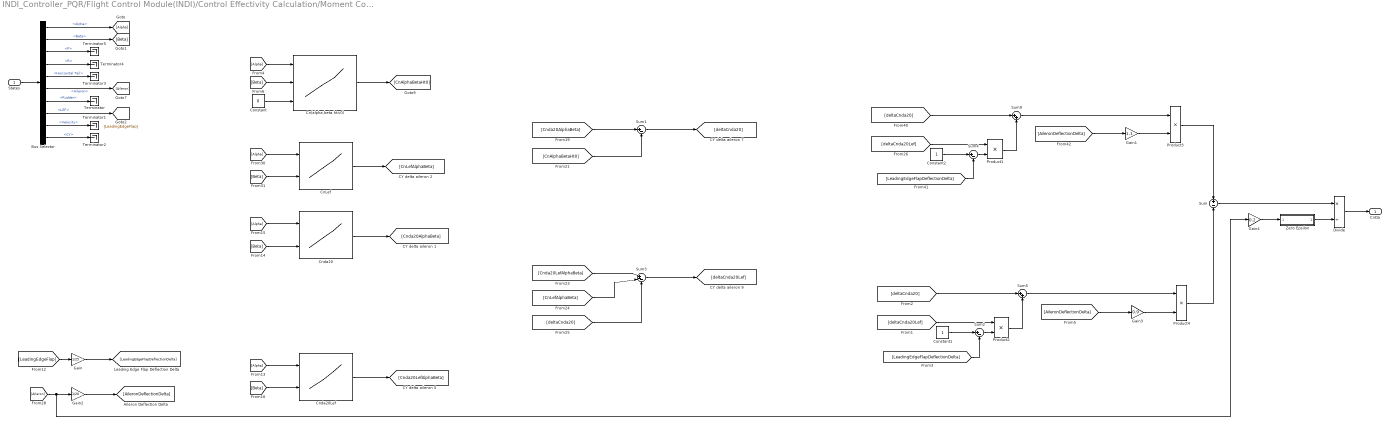
== system INDI_Controller_PQR/Flight Control Module(INDI)/Control Effectivity Calculation/Moment Coeffs/Yaw Moment1 ==
  States : Inport
  Bus Selector : BusSelector  OutputSignals=Alpha,Beta,P,R,Horizontal Tail,Aileron,Rudder,LEF,Velocity,CY
  Cn(alpha,beta,ht=0) : Lookup_n-D  NumberOfTableDimensions=3  BreakpointsForDimension1=dataBase.f16_AerodynamicData.BP.Cn.Cn.alpha  BreakpointsForDimension2=dataBase.f16_AerodynamicData.BP.Cn.Cn.beta  BreakpointsForDimension3=dataBase.f16_AerodynamicData.BP.Cn.Cn.dHT  Table=dataBase.f16_AerodynamicData.data.Cn.Cn  ExtrapMethod=Clip  InternalRulePriority=Speed  RndMeth=Simplest
      settings: InputPortMap=u0,u1,u2
  CnLef : Lookup_n-D  BreakpointsForDimension1=dataBase.f16_AerodynamicData.BP.Cn.Cnlef.alpha  BreakpointsForDimension2=dataBase.f16_AerodynamicData.BP.Cn.Cnlef.beta  Table=dataBase.f16_AerodynamicData.data.Cn.Cnlef  ExtrapMethod=Clip  InternalRulePriority=Speed  RndMeth=Simplest
      settings: InputPortMap=u0,u1
  Cnda20 : Lookup_n-D  BreakpointsForDimension1=dataBase.f16_AerodynamicData.BP.Cn.Cnda20.alpha  BreakpointsForDimension2=dataBase.f16_AerodynamicData.BP.Cn.Cnda20.beta  Table=dataBase.f16_AerodynamicData.data.Cn.Cnda20  ExtrapMethod=Clip  InternalRulePriority=Speed  RndMeth=Simplest
      settings: InputPortMap=u0,u1
  Cnda20Lef : Lookup_n-D  BreakpointsForDimension1=dataBase.f16_AerodynamicData.BP.Cn.Cnda20lef.alpha  BreakpointsForDimension2=dataBase.f16_AerodynamicData.BP.Cn.Cnda20lef.beta  Table=dataBase.f16_AerodynamicData.data.Cn.Cnda20lef  ExtrapMethod=Clip  InternalRulePriority=Speed  RndMeth=Simplest
      settings: InputPortMap=u0,u1
  Constant : Constant  Value=0
  Constant1 : Constant
  Constant2 : Constant
  Divide : Product  Inputs=*/
  Gain : Gain  Gain=1/25
  Gain1 : Gain  Gain=1.1
  Gain2 : Gain  Gain=1/20
  Gain3 : Gain  Gain=0.9
  Gain4 : Gain  Gain=0.2
  Product{1..4} (4 alike) : Product
  Sum : Sum  Inputs=+|-
  Sum1 : Sum  Inputs=|+-
  Sum2 : Sum  Inputs=|+-
  Sum3 : Sum  Inputs=|+--
  Sum4 : Sum  Inputs=|+-
  Sum5 : Sum  Inputs=|++
  Sum9 : Sum  Inputs=|++
  Terminator{,1..5} (6 alike) : Terminator
  Zero Epsilon : Subsystem  ReferencedSubsystem=Zero_Epsilon
  CnDa : Outport
  wires:
  Zero Epsilon/1 -> Divide/2
  Gain4/1 -> Zero Epsilon/1
  States/1 -> Bus Selector/1
  [LeadingEdgeFlap] -> Gain/1
  Gain2/1 -> [AileronDeflectionDelta]
  [Aileron] -> Gain4/1, Gain2/1
  Gain/1 -> [LeadingEdgeFlapDeflectionDelta]
  Cn(alpha,beta,ht=0)/1 -> [CnAlphaBetaHt0]
  [Beta] -> Cn(alpha,beta,ht=0)/2
  [Alpha] -> Cn(alpha,beta,ht=0)/1
  Constant/1 -> Cn(alpha,beta,ht=0)/3
  [Beta] -> CnLef/2
  CnLef/1 -> [CnLefAlphaBeta]
  [Alpha] -> CnLef/1
  [Alpha] -> Cnda20/1
  [Beta] -> Cnda20/2
  Cnda20/1 -> [Cnda20AlphaBeta]
  Cnda20Lef/1 -> [Cnda20LefAlphaBeta]
  [Beta] -> Cnda20Lef/2
  [Alpha] -> Cnda20Lef/1
  Sum1/1 -> [deltaCnda20]
  [CnAlphaBetaHt0] -> Sum1/2
  [Cnda20AlphaBeta] -> Sum1/1
  [Cnda20LefAlphaBeta] -> Sum3/1
  [CnLefAlphaBeta] -> Sum3/2
  [deltaCnda20] -> Sum3/3
  Sum3/1 -> [deltaCnda20Lef]
  Product1/1 -> Sum9/2
  Constant2/1 -> Sum4/1
  Sum4/1 -> Product1/2
  [LeadingEdgeFlapDeflectionDelta] -> Sum4/2
  Sum9/1 -> Product3/1
  [deltaCnda20] -> Sum9/1
  [deltaCnda20Lef] -> Product1/1
  Bus Selector/1 -> [Alpha]  "<Alpha>"
  Bus Selector/2 -> [Beta]  "<Beta>"
  Bus Selector/4 -> Terminator4/1  "<R>"
  Bus Selector/3 -> Terminator5/1  "<P>"
  Bus Selector/5 -> Terminator3/1  "<Horizontal Tail>"
  Bus Selector/6 -> [Aileron]  "<Aileron>"
  Bus Selector/8 -> [LeadingEdgeFlap]  "<LEF>"
  Bus Selector/10 -> Terminator2/1  "<CY>"
  [AileronDeflectionDelta] -> Gain1/1
  Gain1/1 -> Product3/2
  Product3/1 -> Sum/1
  Product4/1 -> Sum/2
  Sum2/1 -> Product2/2
  [deltaCnda20] -> Sum5/1
  Constant1/1 -> Sum2/1
  [LeadingEdgeFlapDeflectionDelta] -> Sum2/2
  Sum5/1 -> Product4/1
  Product2/1 -> Sum5/2
  [AileronDeflectionDelta] -> Gain3/1
  Gain3/1 -> Product4/2
  [deltaCnda20Lef] -> Product2/1
  Sum/1 -> Divide/1
  Divide/1 -> CnDa/1
  Bus Selector/7 -> Terminator/1  "<Rudder>"
  Bus Selector/9 -> Terminator1/1  "<Velocity>"

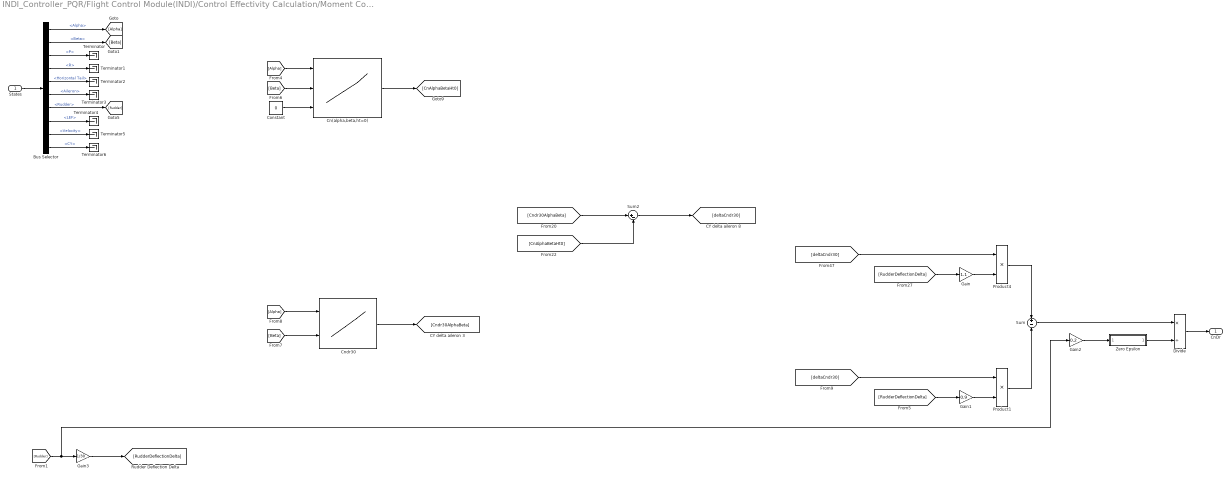
== system INDI_Controller_PQR/Flight Control Module(INDI)/Control Effectivity Calculation/Moment Coeffs/Yaw Moment2 ==
  States : Inport
  Bus Selector : BusSelector  OutputSignals=Alpha,Beta,P,R,Horizontal Tail,Aileron,Rudder,LEF,Velocity,CY
  Cn(alpha,beta,ht=0) : Lookup_n-D  NumberOfTableDimensions=3  BreakpointsForDimension1=dataBase.f16_AerodynamicData.BP.Cn.Cn.alpha  BreakpointsForDimension2=dataBase.f16_AerodynamicData.BP.Cn.Cn.beta  BreakpointsForDimension3=dataBase.f16_AerodynamicData.BP.Cn.Cn.dHT  Table=dataBase.f16_AerodynamicData.data.Cn.Cn  ExtrapMethod=Clip  InternalRulePriority=Speed  RndMeth=Simplest
      settings: InputPortMap=u0,u1,u2
  Cndr30 : Lookup_n-D  BreakpointsForDimension1=dataBase.f16_AerodynamicData.BP.Cn.Cndr30.alpha  BreakpointsForDimension2=dataBase.f16_AerodynamicData.BP.Cn.Cndr30.beta  Table=dataBase.f16_AerodynamicData.data.Cn.Cndr30  ExtrapMethod=Clip  InternalRulePriority=Speed  RndMeth=Simplest
      settings: InputPortMap=u0,u1
  Constant : Constant  Value=0
  Divide : Product  Inputs=*/
  Gain : Gain  Gain=1.1
  Gain1 : Gain  Gain=0.9
  Gain2 : Gain  Gain=0.2
  Gain3 : Gain  Gain=1/30
  Product1 : Product
  Product4 : Product
  Sum : Sum  Inputs=+|-
  Sum2 : Sum  Inputs=|+-
  Terminator{,1..6} (7 alike) : Terminator
  Zero Epsilon : Subsystem  ReferencedSubsystem=Zero_Epsilon
  CnDr : Outport
  wires:
  Zero Epsilon/1 -> Divide/2
  Gain2/1 -> Zero Epsilon/1
  States/1 -> Bus Selector/1
  [Rudder] -> Gain2/1, Gain3/1
  Gain3/1 -> [RudderDeflectionDelta]
  Cn(alpha,beta,ht=0)/1 -> [CnAlphaBetaHt0]
  [Beta] -> Cn(alpha,beta,ht=0)/2
  [Alpha] -> Cn(alpha,beta,ht=0)/1
  Constant/1 -> Cn(alpha,beta,ht=0)/3
  Cndr30/1 -> [Cndr30AlphaBeta]
  [Beta] -> Cndr30/2
  [Alpha] -> Cndr30/1
  [Cndr30AlphaBeta] -> Sum2/1
  [CnAlphaBetaHt0] -> Sum2/2
  Sum2/1 -> [deltaCndr30]
  [deltaCndr30] -> Product4/1
  Bus Selector/1 -> [Alpha]  "<Alpha>"
  Bus Selector/2 -> [Beta]  "<Beta>"
  Bus Selector/3 -> Terminator/1  "<P>"
  Bus Selector/5 -> Terminator2/1  "<Horizontal Tail>"
  Bus Selector/6 -> Terminator3/1  "<Aileron>"
  Bus Selector/7 -> [Rudder]  "<Rudder>"
  Bus Selector/8 -> Terminator4/1  "<LEF>"
  Bus Selector/10 -> Terminator6/1  "<CY>"
  [RudderDeflectionDelta] -> Gain/1
  Gain/1 -> Product4/2
  Product4/1 -> Sum/1
  Product1/1 -> Sum/2
  Gain1/1 -> Product1/2
  [RudderDeflectionDelta] -> Gain1/1
  [deltaCndr30] -> Product1/1
  Sum/1 -> Divide/1
  Divide/1 -> CnDr/1
  Bus Selector/9 -> Terminator5/1  "<Velocity>"
  Bus Selector/4 -> Terminator1/1  "<R>"
